simulink model "AFE_artificial"  (R2019b)
settings: Solver=FixedStepAuto  StartTime=0.0  StopTime=10.0  FixedStep=fixedStepSize  RelTol=1e-3
undefined symbols (not defined in the file): AFE_downThreshold, AFE_speedMin, AFE_subsystem1_downThreshold, AFE_subsystem1_gear, AFE_subsystem1_gearSelectionState, AFE_subsystem1_notAlwaysTimeHorizon, AFE_subsystem1_upThreshold1, AFE_subsystem1_upThreshold2, artificial_AFE_RFC_constant, artificial_AOT_AFE_constant, fixedStepSize
settings Model: Creator=JEDDELAN  LastModifiedBy=JEDDELAN
settings DataIOCC: SaveOutput=off  SaveTime=off  ReturnWorkspaceOutputs=off
settings DebuggingCC: ArithmeticOperatorsInVariantConditions=warning
settings SFSimCC: SimUseLocalCustomCode=off  CustomCodeUndefinedFunction=UseInterfaceOnly
settings RTWCC: RTWUseLocalCustomCode=off
settings GRTTargetCC: CombineOutputUpdateFcns=off  MatFileLogging=off

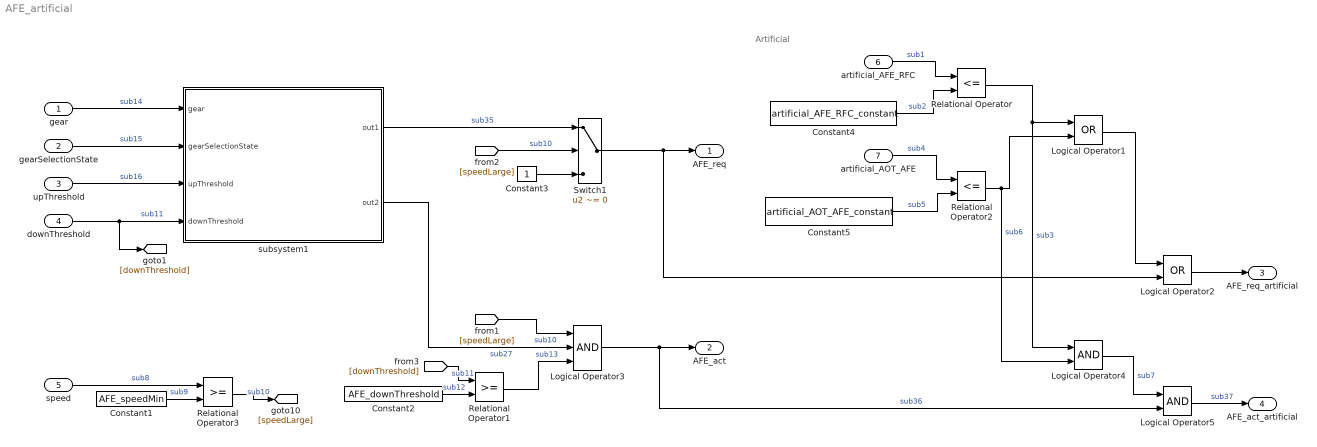
== system AFE_artificial ==
  note: Artificial
  gear : Inport
  gearSelectionState : Inport  Port=2
  upThreshold : Inport  Port=3
  downThreshold : Inport  Port=4
  speed : Inport  Port=5
  artificial_AFE_RFC : Inport  Port=6
  artificial_AOT_AFE : Inport  Port=7
  Constant1 : Constant  Value=AFE_speedMin
  Constant2 : Constant  Value=AFE_downThreshold
  Constant3 : Constant
  Constant4 : Constant  Value=artificial_AFE_RFC_constant
  Constant5 : Constant  Value=artificial_AOT_AFE_constant
  Logical Operator1 : Logic  Operator=OR  AllPortsSameDT=off  OutDataTypeStr=boolean
  Logical Operator2 : Logic  Operator=OR  AllPortsSameDT=off  OutDataTypeStr=boolean
  Logical Operator3 : Logic  Inputs=3  AllPortsSameDT=off  OutDataTypeStr=boolean
  Logical Operator4 : Logic  AllPortsSameDT=off  OutDataTypeStr=boolean
  Logical Operator5 : Logic  AllPortsSameDT=off  OutDataTypeStr=boolean
  Relational Operator : RelationalOperator  Operator=<=  OutDataTypeStr=boolean  RndMeth=Simplest
  Relational Operator1 : RelationalOperator  OutDataTypeStr=boolean  RndMeth=Nearest
  Relational Operator2 : RelationalOperator  Operator=<=  OutDataTypeStr=boolean  RndMeth=Simplest
  Relational Operator3 : RelationalOperator  OutDataTypeStr=boolean  RndMeth=Nearest
  Switch1 : Switch  Criteria=u2 ~= 0
  subsystem1 : Subsystem
  AFE_req : Outport  OutDataTypeStr=boolean  PortDimensions=1  VectorParamsAs1DForOutWhenUnconnected=off
  AFE_act : Outport  Port=2  OutDataTypeStr=boolean  PortDimensions=1  VectorParamsAs1DForOutWhenUnconnected=off
  AFE_req_artificial : Outport  Port=3  OutDataTypeStr=boolean  PortDimensions=1  VectorParamsAs1DForOutWhenUnconnected=off
  AFE_act_artificial : Outport  Port=4  OutDataTypeStr=boolean  PortDimensions=1  VectorParamsAs1DForOutWhenUnconnected=off
  wires:
  Relational Operator3/1 -> [speedLarge]  "sub10"
  Constant3/1 -> Switch1/3
  Constant1/1 -> Relational Operator3/2  "sub9"
  Constant2/1 -> Relational Operator1/2  "sub12"
  [speedLarge] -> Switch1/2  "sub10"
  Relational Operator1/1 -> Logical Operator3/3  "sub13"
  downThreshold/1 -> subsystem1/4(downThreshold), [downThreshold]  "sub11"
  upThreshold/1 -> subsystem1/3(upThreshold)  "sub16"
  subsystem1/2(out2) -> Logical Operator3/2  "sub27"
  subsystem1/1(out1) -> Switch1/1  "sub35"
  [speedLarge] -> Logical Operator3/1  "sub10"
  gearSelectionState/1 -> subsystem1/2(gearSelectionState)  "sub15"
  gear/1 -> subsystem1/1(gear)  "sub14"
  [downThreshold] -> Relational Operator1/1  "sub11"
  speed/1 -> Relational Operator3/1  "sub8"
  Constant4/1 -> Relational Operator/2  "sub2"
  Switch1/1 -> Logical Operator2/2, AFE_req/1
  Logical Operator5/1 -> AFE_act_artificial/1  "sub37"
  Logical Operator4/1 -> Logical Operator5/1  "sub7"
  Relational Operator2/1 -> Logical Operator4/2, Logical Operator1/2  "sub6"
  Constant5/1 -> Relational Operator2/2  "sub5"
  Relational Operator/1 -> Logical Operator4/1, Logical Operator1/1  "sub3"
  artificial_AOT_AFE/1 -> Relational Operator2/1  "sub4"
  Logical Operator1/1 -> Logical Operator2/1
  Logical Operator3/1 -> Logical Operator5/2, AFE_act/1  "sub36"
  Logical Operator2/1 -> AFE_req_artificial/1
  artificial_AFE_RFC/1 -> Relational Operator/1  "sub1"

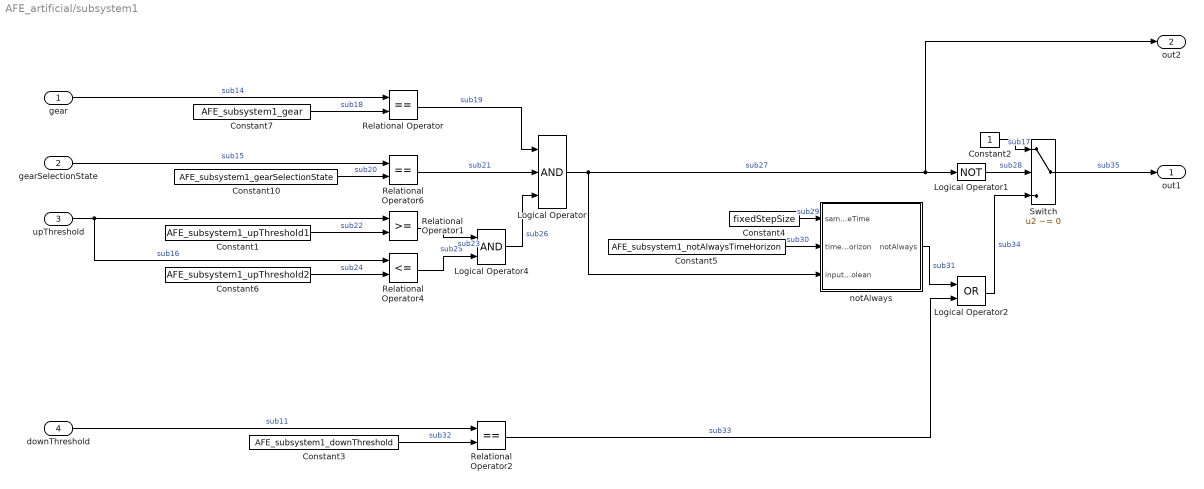
== system AFE_artificial/subsystem1 ==
  gear : Inport
  gearSelectionState : Inport  Port=2
  upThreshold : Inport  Port=3
  downThreshold : Inport  Port=4
  Constant1 : Constant  Value=AFE_subsystem1_upThreshold1
  Constant10 : Constant  Value=AFE_subsystem1_gearSelectionState
  Constant2 : Constant
  Constant3 : Constant  Value=AFE_subsystem1_downThreshold
  Constant4 : Constant  Value=fixedStepSize
  Constant5 : Constant  Value=AFE_subsystem1_notAlwaysTimeHorizon
  Constant6 : Constant  Value=AFE_subsystem1_upThreshold2
  Constant7 : Constant  Value=AFE_subsystem1_gear
  Logical Operator : Logic  Inputs=3  AllPortsSameDT=off  OutDataTypeStr=boolean
  Logical Operator1 : Logic  Operator=NOT  Inputs=3  AllPortsSameDT=off  OutDataTypeStr=boolean
  Logical Operator2 : Logic  Operator=OR  AllPortsSameDT=off  OutDataTypeStr=boolean
  Logical Operator4 : Logic  AllPortsSameDT=off  OutDataTypeStr=boolean
  Relational Operator : RelationalOperator  Operator===  OutDataTypeStr=boolean  RndMeth=Nearest
  Relational Operator1 : RelationalOperator  OutDataTypeStr=boolean  RndMeth=Nearest
  Relational Operator2 : RelationalOperator  Operator===  OutDataTypeStr=boolean  RndMeth=Nearest
  Relational Operator4 : RelationalOperator  Operator=<=  OutDataTypeStr=boolean  RndMeth=Nearest
  Relational Operator6 : RelationalOperator  Operator===  OutDataTypeStr=boolean  RndMeth=Nearest
  Switch : Switch  Criteria=u2 ~= 0
  notAlways : Subsystem
      settings: CopyFcn=set_param(gcbh,'LinkStatus','none');
  out1 : Outport  VectorParamsAs1DForOutWhenUnconnected=off
  out2 : Outport  Port=2  VectorParamsAs1DForOutWhenUnconnected=off
  wires:
  Logical Operator4/1 -> Logical Operator/3  "sub26"
  Relational Operator4/1 -> Logical Operator4/2  "sub25"
  Constant6/1 -> Relational Operator4/2  "sub24"
  gear/1 -> Relational Operator/1  "sub14"
  Constant7/1 -> Relational Operator/2  "sub18"
  Relational Operator/1 -> Logical Operator/1  "sub19"
  gearSelectionState/1 -> Relational Operator6/1  "sub15"
  upThreshold/1 -> Relational Operator1/1, Relational Operator4/1  "sub16"
  Constant1/1 -> Relational Operator1/2  "sub22"
  Relational Operator1/1 -> Logical Operator4/1  "sub23"
  Logical Operator/1 -> notAlways/3(inputBoolean), Logical Operator1/1, out2/1  "sub27"
  Constant2/1 -> Switch/1  "sub17"
  downThreshold/1 -> Relational Operator2/1  "sub11"
  Constant3/1 -> Relational Operator2/2  "sub32"
  Relational Operator2/1 -> Logical Operator2/2  "sub33"
  notAlways/1(notAlways) -> Logical Operator2/1  "sub31"
  Logical Operator2/1 -> Switch/3  "sub34"
  Constant4/1 -> notAlways/1(sampleTime)  "sub29"
  Constant5/1 -> notAlways/2(timeHorizon)  "sub30"
  Switch/1 -> out1/1  "sub35"
  Logical Operator1/1 -> Switch/2  "sub28"
  Constant10/1 -> Relational Operator6/2  "sub20"
  Relational Operator6/1 -> Logical Operator/2  "sub21"

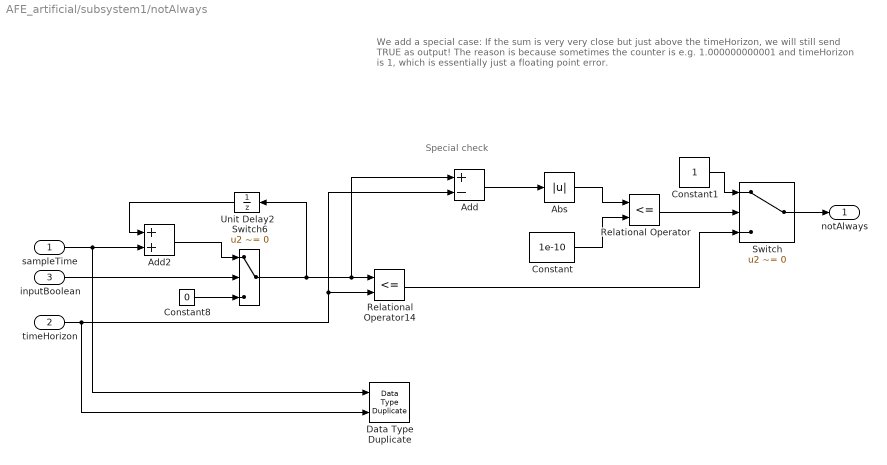
== system AFE_artificial/subsystem1/notAlways ==
  note: Special check
  note: We add a special case:
      | If the sum is very very close but just above the timeHorizon, we will still send TRUE as output!
      |
      | The reason is because sometimes the counter is e.g. 1.000000000001 and timeHorizon is 1, which is essentially just a floating point error.
  sampleTime : Inport
  timeHorizon : Inport  Port=2
  inputBoolean : Inport  Port=3
  Abs : Abs
  Add : Sum  Inputs=+-
  Add2 : Sum
  Constant : Constant  Value=1e-10
  Constant1 : Constant  OutDataTypeStr=boolean
  Constant8 : Constant  Value=0  OutDataTypeStr=Inherit: Inherit via back propagation
  Data Type Duplicate : DataTypeDuplicate
  Relational Operator : RelationalOperator  Operator=<=  OutDataTypeStr=boolean  RndMeth=Simplest
  Relational Operator14 : RelationalOperator  Operator=<=  OutDataTypeStr=boolean  RndMeth=Nearest
  Switch : Switch  Criteria=u2 ~= 0
  Switch6 : Switch  Criteria=u2 ~= 0
  Unit Delay2 : UnitDelay  SampleTime=-1  HasFrameUpgradeWarning=on
  notAlways : Outport  VectorParamsAs1DForOutWhenUnconnected=off
  wires:
  Switch6/1 -> Add/1, Relational Operator14/1, Unit Delay2/1
  timeHorizon/1 -> Add/2, Relational Operator14/2, Data Type Duplicate/2
  Relational Operator14/1 -> Switch/3
  Unit Delay2/1 -> Add2/1
  Add2/1 -> Switch6/1
  sampleTime/1 -> Add2/2, Data Type Duplicate/1
  Constant8/1 -> Switch6/3
  inputBoolean/1 -> Switch6/2
  Add/1 -> Abs/1
  Abs/1 -> Relational Operator/1
  Constant/1 -> Relational Operator/2
  Relational Operator/1 -> Switch/2
  Constant1/1 -> Switch/1
  Switch/1 -> notAlways/1
